simulink model "continuous"  (R2015a)
settings: Solver=ode45  StartTime=0.0  StopTime=10.0  RelTol=1e-3
settings Model: Creator=theth  LastModifiedBy=theth

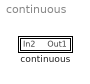
== system continuous ==
  continuous : Subsystem

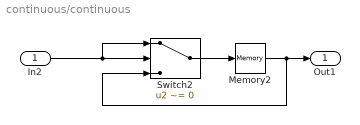
== system continuous/continuous ==
  In2 : Inport
  Memory2 : Memory
  Switch2 : Switch  Criteria=u2 ~= 0
  Out1 : Outport
  wires:
  Memory2/1 -> Switch2/3, Out1/1
  Switch2/1 -> Memory2/1
  In2/1 -> Switch2/1, Switch2/2
